simulink model "friction_model_comparison_Roldasfucka"  (R2014a)
settings: Solver=ode45  SolverMode=SingleTasking  StartTime=0.0  StopTime=8  MaxStep=1e-6  RelTol=1e-3
libraries: simulink x2
settings Model: CovMetricSettings=dwe  CovHtmlReporting=off  covSaveCumulativeToWorkspaceVar=off  CovSaveSingleToWorkspaceVar=off  CovExternalEMLEnable=on  CovSFcnEnable=on  Creator=Charlie  LastModifiedBy=Charlie
settings SolverCC: MaxConsecutiveZCs=1e6  ZeroCrossAlgorithm=Adaptive
settings DataIOCC: LimitDataPoints=off  SaveFormat=StructureWithTime  ReturnWorkspaceOutputs=on
settings DebuggingCC: MergeDetectMultiDrivingBlocksExec=error  SolverPrmCheckMsg=none  FrameProcessingCompatibilityMsg=error  SFUnexpectedBacktrackingDiag=error  SFNoUnconditionalDefaultTransitionDiag=error
settings HardwareCC: ProdBitPerPointer=64  ProdLargestAtomicFloat=Float  ProdIntDivRoundTo=Zero  ProdEndianess=LittleEndian  ProdHWDeviceType=Specified
settings ModelReferenceCC: PropagateSignalLabelsOutOfModel=on
settings SFSimCC: SimUseLocalCustomCode=on
settings RTWCC: RTWUseLocalCustomCode=on
settings GRTTargetCC: TargetLangStandard=C99 (ISO)

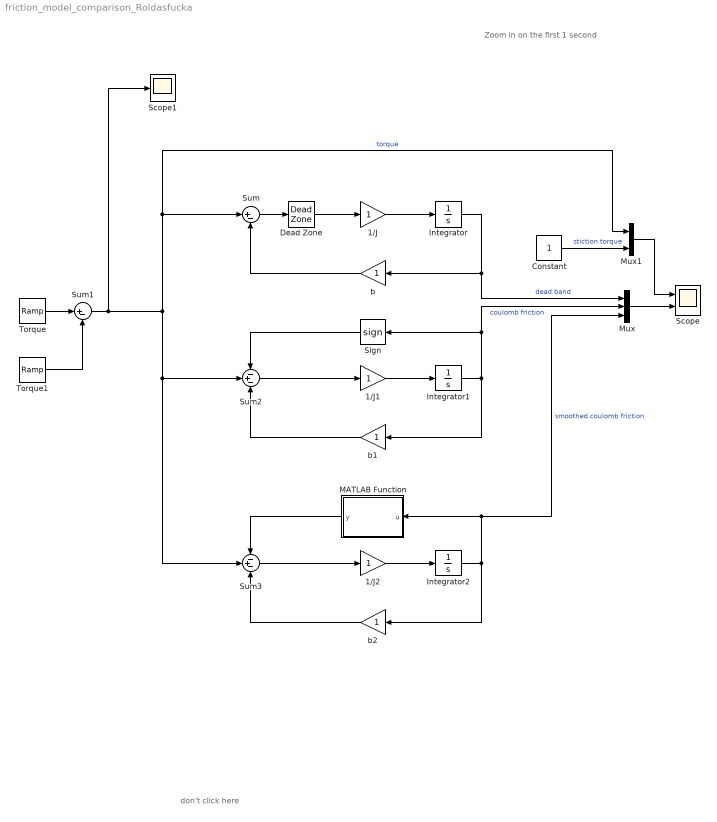
== system friction_model_comparison_Roldasfucka ==
  note: don't click here
  note: Zoom in on the first 1 second
  1/J : Gain
  1/J1 : Gain
  1/J2 : Gain
  Constant : Constant
  Dead Zone : DeadZone  LowerValue=-1  UpperValue=1  SaturateOnIntegerOverflow=on
  Integrator : Integrator
  Integrator1 : Integrator
  Integrator2 : Integrator
  MATLAB Function : MATLAB Function  TreatAsAtomicUnit=on
      settings: PermitHierarchicalResolution=ParametersOnly
  Mux : Mux  Inputs=3
  Mux1 : Mux  Inputs=2
  Scope : Scope  NumInputPorts=2
      settings: TimeRange=auto  ShowLegends=on  MaxDataPoints=5000  SaveToWorkspace=off  SaveName=ScopeData  YMin=-0.25~-0.12481  YMax=2.25~1.12324  SampleTime=-1
  Scope1 : Scope
      settings: TimeRange=auto  MaxDataPoints=5000  SaveToWorkspace=off  YMin=-0.25  YMax=2.25  SampleTime=-1
  Sign : Signum
  Sum : Sum  Inputs=|+-
  Sum1 : Sum  Inputs=|+-
  Sum2 : Sum  Inputs=-+-
  Sum3 : Sum  Inputs=-+-
  Torque : simulink/Sources/Ramp  slope=1  start=0  X0=0
  Torque1 : simulink/Sources/Ramp  slope=1  start=2  X0=0
  b : Gain
  b1 : Gain
  b2 : Gain
  wires:
  Sum/1 -> Dead Zone/1
  1/J/1 -> Integrator/1
  Dead Zone/1 -> 1/J/1
  Integrator/1 -> Mux/1, b/1  "dead band"
  b/1 -> Sum/2
  Torque/1 -> Sum1/1
  Torque1/1 -> Sum1/2
  b1/1 -> Sum2/3
  Sum2/1 -> 1/J1/1
  1/J1/1 -> Integrator1/1
  Sign/1 -> Sum2/1
  Integrator1/1 -> Mux/2, Sign/1, b1/1  "coulomb friction"
  Integrator2/1 -> b2/1, Mux/3, MATLAB Function/1(u)  "smoothed coulomb friction"
  MATLAB Function/1(y) -> Sum3/1
  1/J2/1 -> Integrator2/1
  Sum3/1 -> 1/J2/1
  b2/1 -> Sum3/3
  Sum1/1 -> Scope1/1, Mux1/1, Sum/1, Sum3/2, Sum2/2  "torque"
  Mux/1 -> Scope/2
  Constant/1 -> Mux1/2  "stiction torque"
  Mux1/1 -> Scope/1

== matlab function friction_model_comparison_Roldasfucka/MATLAB Function ==
  data: u input; y output
function y = fcn(u)

y = erf(1e6*u);
